simulink model "RunningLEDExample"  (R2015a)
settings: Solver=ode3  SolverMode=SingleTasking  StartTime=0.0  StopTime=inf  FixedStep=Ts  RelTol=1e-3
undefined symbols (not defined in the file): Ts
libraries: simulink x1
(part 1 of 2)
settings Model: ExtModeTrigDuration=2  Creator=kkhoo  LastModifiedBy=kkhoo
settings OptimizationCC: OptimizeModelRefInitCode=on  LifeSpan=1
settings DebuggingCC: UnderspecifiedInitializationDetection=Classic  MergeDetectMultiDrivingBlocksExec=none
settings HardwareCC: ProdBitPerInt=16  ProdBitPerPointer=8  ProdIntDivRoundTo=Zero  ProdEndianess=LittleEndian  ProdWordSize=8  ProdHWDeviceType=Atmel->AVR
settings RTWCC: SystemTargetFile=realtime.tlc  GenerateMakefile=off  TemplateMakefile=realtime.tmf  Description=Run on Target Hardware  RTWVerbose=off  CustomSource=src/Engduino.h src/engduino_wrappers.cpp
settings ERTTargetCC: CombineOutputUpdateFcns=off  ExtModeTransport=3  ExtModeMexFile=ext_serial_win32_comm_rtt  ExtModeMexArgs=0 1 9600  ERTSrcFileBannerTemplate=realtime_code_template.cgt  ERTHdrFileBannerTemplate=realtime_code_template.cgt  ERTDataSrcFileTemplate=realtime_code_template.cgt  ERTDataHdrFileTemplate=realtime_code_template.cgt  ERTCustomFileTemplate=realtime_file_process.tlc

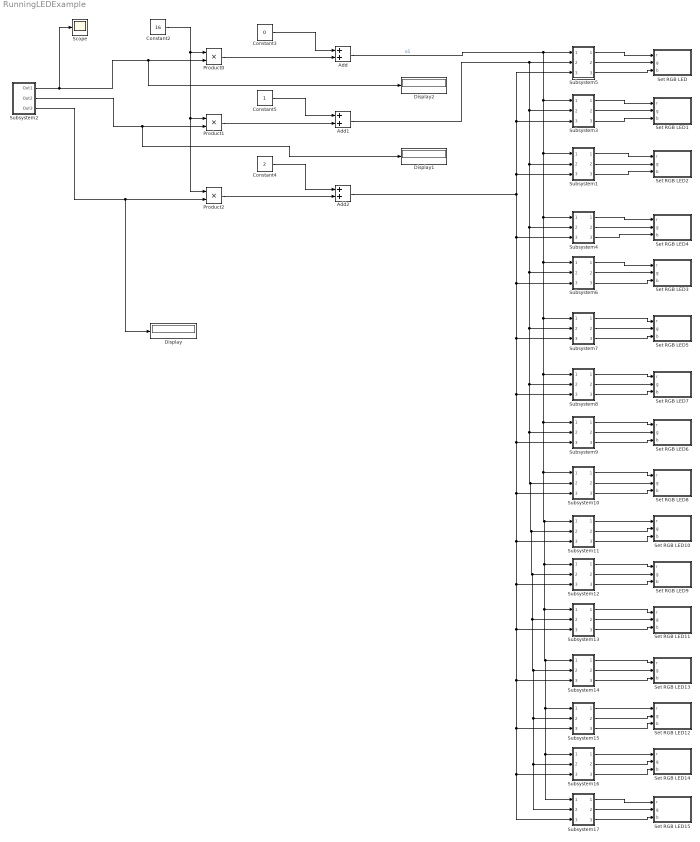
== system RunningLEDExample ==
  Add : Sum  AccumDataTypeStr=single
  Add1 : Sum  AccumDataTypeStr=single
  Add2 : Sum  AccumDataTypeStr=single
  Constant2 : Constant  Value=16  OutDataTypeStr=double
  Constant3 : Constant  Value=0  OutDataTypeStr=single
  Constant4 : Constant  Value=2  OutDataTypeStr=double
  Constant5 : Constant  OutDataTypeStr=double
  Display : Display
  Display1 : Display
  Display2 : Display
  "Product0 " : Product  OutDataTypeStr=double
  Product1 : Product  OutDataTypeStr=double
  Product2 : Product  OutDataTypeStr=double  InputSameDT=on
  Scope : Scope
      settings: YMin=0  YMax=15
  Set RGB LED : MATLAB Function  LoadFcn=|  TreatAsAtomicUnit=on  mask(RGB LED){led_index=0}
      | set_param(gcs, 'CustomSource', strjoin(unique([strsplit(get_param(gcs, 'CustomSource')) ...
      |  'src/engduino_wrappers.cpp' 'src/Engduino.h'])));
      mask prompts: led_index "LED index"
      mask help:
      | Control the Red, Green and Blue color values of the LED specified by the LED index parameter.
      | Both the LED index and the three color values are of type uint8 and must be in the range 0-15.
      settings: AttributesFormatString=LED %<led_index>
  Set RGB LED1 : MATLAB Function  LoadFcn=|  TreatAsAtomicUnit=on  mask(RGB LED){led_index=1}
      | set_param(gcs, 'CustomSource', strjoin(unique([strsplit(get_param(gcs, 'CustomSource')) ...
      |  'src/engduino_wrappers.cpp' 'src/Engduino.h'])));
      mask prompts: led_index "LED index"
      mask help:
      | Control the Red, Green and Blue color values of the LED specified by the LED index parameter.
      | Both the LED index and the three color values are of type uint8 and must be in the range 0-15.
      settings: AttributesFormatString=LED %<led_index>
  Set RGB LED10 : MATLAB Function  LoadFcn=|  TreatAsAtomicUnit=on  mask(RGB LED){led_index=9}
      | set_param(gcs, 'CustomSource', strjoin(unique([strsplit(get_param(gcs, 'CustomSource')) ...
      |  'src/engduino_wrappers.cpp' 'src/Engduino.h'])));
      mask prompts: led_index "LED index"
      mask help:
      | Control the Red, Green and Blue color values of the LED specified by the LED index parameter.
      | Both the LED index and the three color values are of type uint8 and must be in the range 0-15.
      settings: AttributesFormatString=LED %<led_index>
  Set RGB LED11 : MATLAB Function  LoadFcn=|  TreatAsAtomicUnit=on  mask(RGB LED){led_index=11}
      | set_param(gcs, 'CustomSource', strjoin(unique([strsplit(get_param(gcs, 'CustomSource')) ...
      |  'src/engduino_wrappers.cpp' 'src/Engduino.h'])));
      mask prompts: led_index "LED index"
      mask help:
      | Control the Red, Green and Blue color values of the LED specified by the LED index parameter.
      | Both the LED index and the three color values are of type uint8 and must be in the range 0-15.
      settings: AttributesFormatString=LED %<led_index>
  Set RGB LED12 : MATLAB Function  LoadFcn=|  TreatAsAtomicUnit=on  mask(RGB LED){led_index=13}
      | set_param(gcs, 'CustomSource', strjoin(unique([strsplit(get_param(gcs, 'CustomSource')) ...
      |  'src/engduino_wrappers.cpp' 'src/Engduino.h'])));
      mask prompts: led_index "LED index"
      mask help:
      | Control the Red, Green and Blue color values of the LED specified by the LED index parameter.
      | Both the LED index and the three color values are of type uint8 and must be in the range 0-15.
      settings: AttributesFormatString=LED %<led_index>
  Set RGB LED13 : MATLAB Function  LoadFcn=|  TreatAsAtomicUnit=on  mask(RGB LED){led_index=12}
      | set_param(gcs, 'CustomSource', strjoin(unique([strsplit(get_param(gcs, 'CustomSource')) ...
      |  'src/engduino_wrappers.cpp' 'src/Engduino.h'])));
      mask prompts: led_index "LED index"
      mask help:
      | Control the Red, Green and Blue color values of the LED specified by the LED index parameter.
      | Both the LED index and the three color values are of type uint8 and must be in the range 0-15.
      settings: AttributesFormatString=LED %<led_index>
  Set RGB LED14 : MATLAB Function  LoadFcn=|  TreatAsAtomicUnit=on  mask(RGB LED){led_index=14}
      | set_param(gcs, 'CustomSource', strjoin(unique([strsplit(get_param(gcs, 'CustomSource')) ...
      |  'src/engduino_wrappers.cpp' 'src/Engduino.h'])));
      mask prompts: led_index "LED index"
      mask help:
      | Control the Red, Green and Blue color values of the LED specified by the LED index parameter.
      | Both the LED index and the three color values are of type uint8 and must be in the range 0-15.
      settings: AttributesFormatString=LED %<led_index>
  Set RGB LED15 : MATLAB Function  LoadFcn=|  TreatAsAtomicUnit=on  mask(RGB LED){led_index=15}
      | set_param(gcs, 'CustomSource', strjoin(unique([strsplit(get_param(gcs, 'CustomSource')) ...
      |  'src/engduino_wrappers.cpp' 'src/Engduino.h'])));
      mask prompts: led_index "LED index"
      mask help:
      | Control the Red, Green and Blue color values of the LED specified by the LED index parameter.
      | Both the LED index and the three color values are of type uint8 and must be in the range 0-15.
      settings: AttributesFormatString=LED %<led_index>
  Set RGB LED2 : MATLAB Function  LoadFcn=|  TreatAsAtomicUnit=on  mask(RGB LED){led_index=2}
      | set_param(gcs, 'CustomSource', strjoin(unique([strsplit(get_param(gcs, 'CustomSource')) ...
      |  'src/engduino_wrappers.cpp' 'src/Engduino.h'])));
      mask prompts: led_index "LED index"
      mask help:
      | Control the Red, Green and Blue color values of the LED specified by the LED index parameter.
      | Both the LED index and the three color values are of type uint8 and must be in the range 0-15.
      settings: AttributesFormatString=LED %<led_index>
  Set RGB LED3 : MATLAB Function  LoadFcn=|  TreatAsAtomicUnit=on  mask(RGB LED){led_index=4}
      | set_param(gcs, 'CustomSource', strjoin(unique([strsplit(get_param(gcs, 'CustomSource')) ...
      |  'src/engduino_wrappers.cpp' 'src/Engduino.h'])));
      mask prompts: led_index "LED index"
      mask help:
      | Control the Red, Green and Blue color values of the LED specified by the LED index parameter.
      | Both the LED index and the three color values are of type uint8 and must be in the range 0-15.
      settings: AttributesFormatString=LED %<led_index>
  Set RGB LED4 : MATLAB Function  LoadFcn=|  TreatAsAtomicUnit=on  mask(RGB LED){led_index=3}
      | set_param(gcs, 'CustomSource', strjoin(unique([strsplit(get_param(gcs, 'CustomSource')) ...
      |  'src/engduino_wrappers.cpp' 'src/Engduino.h'])));
      mask prompts: led_index "LED index"
      mask help:
      | Control the Red, Green and Blue color values of the LED specified by the LED index parameter.
      | Both the LED index and the three color values are of type uint8 and must be in the range 0-15.
      settings: AttributesFormatString=LED %<led_index>
  Set RGB LED5 : MATLAB Function  LoadFcn=|  TreatAsAtomicUnit=on  mask(RGB LED){led_index=5}
      | set_param(gcs, 'CustomSource', strjoin(unique([strsplit(get_param(gcs, 'CustomSource')) ...
      |  'src/engduino_wrappers.cpp' 'src/Engduino.h'])));
      mask prompts: led_index "LED index"
      mask help:
      | Control the Red, Green and Blue color values of the LED specified by the LED index parameter.
      | Both the LED index and the three color values are of type uint8 and must be in the range 0-15.
      settings: AttributesFormatString=LED %<led_index>
  Set RGB LED6 : MATLAB Function  LoadFcn=|  TreatAsAtomicUnit=on  mask(RGB LED){led_index=7}
      | set_param(gcs, 'CustomSource', strjoin(unique([strsplit(get_param(gcs, 'CustomSource')) ...
      |  'src/engduino_wrappers.cpp' 'src/Engduino.h'])));
      mask prompts: led_index "LED index"
      mask help:
      | Control the Red, Green and Blue color values of the LED specified by the LED index parameter.
      | Both the LED index and the three color values are of type uint8 and must be in the range 0-15.
      settings: AttributesFormatString=LED %<led_index>
  Set RGB LED7 : MATLAB Function  LoadFcn=|  TreatAsAtomicUnit=on  mask(RGB LED){led_index=6}
      | set_param(gcs, 'CustomSource', strjoin(unique([strsplit(get_param(gcs, 'CustomSource')) ...
      |  'src/engduino_wrappers.cpp' 'src/Engduino.h'])));
      mask prompts: led_index "LED index"
      mask help:
      | Control the Red, Green and Blue color values of the LED specified by the LED index parameter.
      | Both the LED index and the three color values are of type uint8 and must be in the range 0-15.
      settings: AttributesFormatString=LED %<led_index>
  Set RGB LED8 : MATLAB Function  LoadFcn=|  TreatAsAtomicUnit=on  mask(RGB LED){led_index=8}
      | set_param(gcs, 'CustomSource', strjoin(unique([strsplit(get_param(gcs, 'CustomSource')) ...
      |  'src/engduino_wrappers.cpp' 'src/Engduino.h'])));
      mask prompts: led_index "LED index"
      mask help:
      | Control the Red, Green and Blue color values of the LED specified by the LED index parameter.
      | Both the LED index and the three color values are of type uint8 and must be in the range 0-15.
      settings: AttributesFormatString=LED %<led_index>
  Set RGB LED9 : MATLAB Function  LoadFcn=|  TreatAsAtomicUnit=on  mask(RGB LED){led_index=10}
      | set_param(gcs, 'CustomSource', strjoin(unique([strsplit(get_param(gcs, 'CustomSource')) ...
      |  'src/engduino_wrappers.cpp' 'src/Engduino.h'])));
      mask prompts: led_index "LED index"
      mask help:
      | Control the Red, Green and Blue color values of the LED specified by the LED index parameter.
      | Both the LED index and the three color values are of type uint8 and must be in the range 0-15.
      settings: AttributesFormatString=LED %<led_index>
  Subsystem1 : Subsystem
  Subsystem10 : Subsystem
  Subsystem11 : Subsystem
  Subsystem12 : Subsystem
  Subsystem13 : Subsystem
  Subsystem14 : Subsystem
  Subsystem15 : Subsystem
  Subsystem16 : Subsystem
  Subsystem17 : Subsystem
  Subsystem2 : Subsystem
  Subsystem3 : Subsystem
  Subsystem4 : Subsystem
  Subsystem5 : Subsystem
  Subsystem6 : Subsystem
  Subsystem7 : Subsystem
  Subsystem8 : Subsystem
  Subsystem9 : Subsystem
  wires:
  Constant2/1 -> "Product0 "/1, Product2/1, Product1/1
  Constant3/1 -> Add/1
  "Product0 "/1 -> Add/2
  Constant5/1 -> Add1/1
  Product1/1 -> Add1/2
  Constant4/1 -> Add2/1
  Product2/1 -> Add2/2
  Subsystem3/1(Out1) -> Set RGB LED1/1(r)
  Subsystem2/1(Out1) -> Scope/1, Display2/1, "Product0 "/2
  Subsystem2/2(Out2) -> Display1/1, Product1/2
  Subsystem2/3(Out3) -> Display/1, Product2/2
  Subsystem5/1(Out1) -> Set RGB LED/1(r)
  Subsystem5/2(Out2) -> Set RGB LED/2(g)
  Subsystem5/3(Out3) -> Set RGB LED/3(b)
  Add/1 -> Subsystem4/1(In1), Subsystem17/1(In1), Subsystem16/1(In1), Subsystem15/1(In1), Subsystem14/1(In1), Subsystem13/1(In1), Subsystem12/1(In1), Subsystem11/1(In1), Subsystem10/1(In1), Subsystem9/1(In1), Subsystem8/1(In1), Subsystem7/1(In1), Subsystem6/1(In1), Subsystem1/1(In1), Subsystem3/1(In1), Subsystem5/1(In1)  "u1"
  Add1/1 -> Subsystem4/2(In2), Subsystem6/2(In2), Subsystem8/2(In2), Subsystem9/2(In2), Subsystem17/2(In2), Subsystem16/2(In2), Subsystem15/2(In2), Subsystem14/2(In2), Subsystem13/2(In2), Subsystem12/2(In2), Subsystem11/2(In2), Subsystem10/2(In2), Subsystem7/2(In2), Subsystem1/2(In2), Subsystem3/2(In2), Subsystem5/2(In2)
  Add2/1 -> Subsystem5/3(In3), Subsystem3/3(In3), Subsystem1/3(In3), Subsystem9/3(In3), Subsystem17/3(In3), Subsystem16/3(In3), Subsystem15/3(In3), Subsystem14/3(In3), Subsystem13/3(In3), Subsystem12/3(In3), Subsystem11/3(In3), Subsystem10/3(In3), Subsystem8/3(In3), Subsystem7/3(In3), Subsystem6/3(In3), Subsystem4/3(In3)
  Subsystem3/2(Out2) -> Set RGB LED1/2(g)
  Subsystem3/3(Out3) -> Set RGB LED1/3(b)
  Subsystem4/1(Out1) -> Set RGB LED4/1(r)
  Subsystem4/2(Out2) -> Set RGB LED4/2(g)
  Subsystem4/3(Out3) -> Set RGB LED4/3(b)
  Subsystem6/1(Out1) -> Set RGB LED3/1(r)
  Subsystem6/2(Out2) -> Set RGB LED3/2(g)
  Subsystem6/3(Out3) -> Set RGB LED3/3(b)
  Subsystem7/1(Out1) -> Set RGB LED5/1(r)
  Subsystem7/2(Out2) -> Set RGB LED5/2(g)
  Subsystem7/3(Out3) -> Set RGB LED5/3(b)
  Subsystem8/1(Out1) -> Set RGB LED7/1(r)
  Subsystem8/2(Out2) -> Set RGB LED7/2(g)
  Subsystem8/3(Out3) -> Set RGB LED7/3(b)
  Subsystem1/1(Out1) -> Set RGB LED2/1(r)
  Subsystem1/2(Out2) -> Set RGB LED2/2(g)
  Subsystem1/3(Out3) -> Set RGB LED2/3(b)
  Subsystem9/1(Out1) -> Set RGB LED6/1(r)
  Subsystem9/2(Out2) -> Set RGB LED6/2(g)
  Subsystem9/3(Out3) -> Set RGB LED6/3(b)
  Subsystem10/1(Out1) -> Set RGB LED8/1(r)
  Subsystem10/2(Out2) -> Set RGB LED8/2(g)
  Subsystem10/3(Out3) -> Set RGB LED8/3(b)
  Subsystem11/1(Out1) -> Set RGB LED10/1(r)
  Subsystem11/2(Out2) -> Set RGB LED10/2(g)
  Subsystem11/3(Out3) -> Set RGB LED10/3(b)
  Subsystem12/1(Out1) -> Set RGB LED9/1(r)
  Subsystem12/2(Out2) -> Set RGB LED9/2(g)
  Subsystem12/3(Out3) -> Set RGB LED9/3(b)
  Subsystem13/1(Out1) -> Set RGB LED11/1(r)
  Subsystem13/2(Out2) -> Set RGB LED11/2(g)
  Subsystem13/3(Out3) -> Set RGB LED11/3(b)
  Subsystem14/2(Out2) -> Set RGB LED13/2(g)
  Subsystem14/1(Out1) -> Set RGB LED13/1(r)
  Subsystem14/3(Out3) -> Set RGB LED13/3(b)
  Subsystem15/1(Out1) -> Set RGB LED12/1(r)
  Subsystem15/2(Out2) -> Set RGB LED12/2(g)
  Subsystem15/3(Out3) -> Set RGB LED12/3(b)
  Subsystem16/1(Out1) -> Set RGB LED14/1(r)
  Subsystem16/2(Out2) -> Set RGB LED14/2(g)
  Subsystem16/3(Out3) -> Set RGB LED14/3(b)
  Subsystem17/1(Out1) -> Set RGB LED15/1(r)
  Subsystem17/2(Out2) -> Set RGB LED15/2(g)
  Subsystem17/3(Out3) -> Set RGB LED15/3(b)

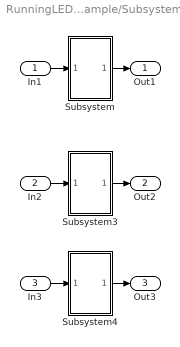
== system RunningLEDExample/Subsystem1 ==
  In1 : Inport
  In2 : Inport  Port=2
  In3 : Inport  Port=3
  Subsystem : Subsystem
  Subsystem3 : Subsystem
  Subsystem4 : Subsystem
  Out1 : Outport
  Out2 : Outport  Port=2
  Out3 : Outport  Port=3
  wires:
  In1/1 -> Subsystem/1(In1)
  Subsystem4/1(Out1) -> Out3/1
  In2/1 -> Subsystem3/1(In1)
  Subsystem/1(Out1) -> Out1/1
  In3/1 -> Subsystem4/1(In1)
  Subsystem3/1(Out1) -> Out2/1

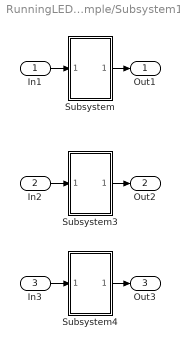
== system RunningLEDExample/Subsystem10 ==
  In1 : Inport
  In2 : Inport  Port=2
  In3 : Inport  Port=3
  Subsystem : Subsystem
  Subsystem3 : Subsystem
  Subsystem4 : Subsystem
  Out1 : Outport
  Out2 : Outport  Port=2
  Out3 : Outport  Port=3
  wires:
  In1/1 -> Subsystem/1(In1)
  Subsystem4/1(Out1) -> Out3/1
  In2/1 -> Subsystem3/1(In1)
  Subsystem/1(Out1) -> Out1/1
  In3/1 -> Subsystem4/1(In1)
  Subsystem3/1(Out1) -> Out2/1

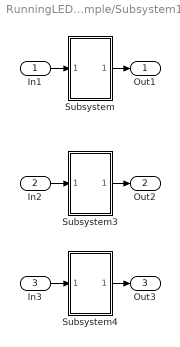
== system RunningLEDExample/Subsystem11 ==
  In1 : Inport
  In2 : Inport  Port=2
  In3 : Inport  Port=3
  Subsystem : Subsystem
  Subsystem3 : Subsystem
  Subsystem4 : Subsystem
  Out1 : Outport
  Out2 : Outport  Port=2
  Out3 : Outport  Port=3
  wires:
  In1/1 -> Subsystem/1(In1)
  Subsystem4/1(Out1) -> Out3/1
  In2/1 -> Subsystem3/1(In1)
  Subsystem/1(Out1) -> Out1/1
  In3/1 -> Subsystem4/1(In1)
  Subsystem3/1(Out1) -> Out2/1

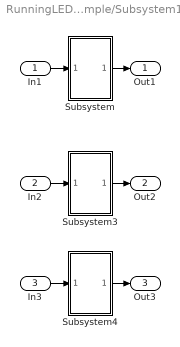
== system RunningLEDExample/Subsystem12 ==
  In1 : Inport
  In2 : Inport  Port=2
  In3 : Inport  Port=3
  Subsystem : Subsystem
  Subsystem3 : Subsystem
  Subsystem4 : Subsystem
  Out1 : Outport
  Out2 : Outport  Port=2
  Out3 : Outport  Port=3
  wires:
  In1/1 -> Subsystem/1(In1)
  Subsystem4/1(Out1) -> Out3/1
  In2/1 -> Subsystem3/1(In1)
  Subsystem/1(Out1) -> Out1/1
  In3/1 -> Subsystem4/1(In1)
  Subsystem3/1(Out1) -> Out2/1

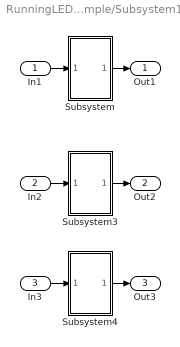
== system RunningLEDExample/Subsystem13 ==
  In1 : Inport
  In2 : Inport  Port=2
  In3 : Inport  Port=3
  Subsystem : Subsystem
  Subsystem3 : Subsystem
  Subsystem4 : Subsystem
  Out1 : Outport
  Out2 : Outport  Port=2
  Out3 : Outport  Port=3
  wires:
  In1/1 -> Subsystem/1(In1)
  Subsystem4/1(Out1) -> Out3/1
  In2/1 -> Subsystem3/1(In1)
  Subsystem/1(Out1) -> Out1/1
  In3/1 -> Subsystem4/1(In1)
  Subsystem3/1(Out1) -> Out2/1

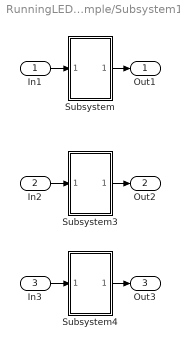
== system RunningLEDExample/Subsystem14 ==
  In1 : Inport
  In2 : Inport  Port=2
  In3 : Inport  Port=3
  Subsystem : Subsystem
  Subsystem3 : Subsystem
  Subsystem4 : Subsystem
  Out1 : Outport
  Out2 : Outport  Port=2
  Out3 : Outport  Port=3
  wires:
  In1/1 -> Subsystem/1(In1)
  Subsystem4/1(Out1) -> Out3/1
  In2/1 -> Subsystem3/1(In1)
  Subsystem/1(Out1) -> Out1/1
  In3/1 -> Subsystem4/1(In1)
  Subsystem3/1(Out1) -> Out2/1

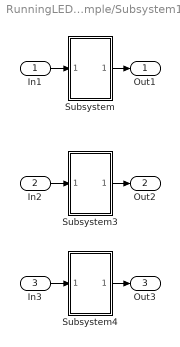
== system RunningLEDExample/Subsystem15 ==
  In1 : Inport
  In2 : Inport  Port=2
  In3 : Inport  Port=3
  Subsystem : Subsystem
  Subsystem3 : Subsystem
  Subsystem4 : Subsystem
  Out1 : Outport
  Out2 : Outport  Port=2
  Out3 : Outport  Port=3
  wires:
  In1/1 -> Subsystem/1(In1)
  Subsystem4/1(Out1) -> Out3/1
  In2/1 -> Subsystem3/1(In1)
  Subsystem/1(Out1) -> Out1/1
  In3/1 -> Subsystem4/1(In1)
  Subsystem3/1(Out1) -> Out2/1

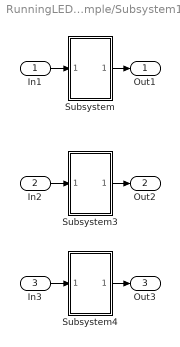
== system RunningLEDExample/Subsystem16 ==
  In1 : Inport
  In2 : Inport  Port=2
  In3 : Inport  Port=3
  Subsystem : Subsystem
  Subsystem3 : Subsystem
  Subsystem4 : Subsystem
  Out1 : Outport
  Out2 : Outport  Port=2
  Out3 : Outport  Port=3
  wires:
  In1/1 -> Subsystem/1(In1)
  Subsystem4/1(Out1) -> Out3/1
  In2/1 -> Subsystem3/1(In1)
  Subsystem/1(Out1) -> Out1/1
  In3/1 -> Subsystem4/1(In1)
  Subsystem3/1(Out1) -> Out2/1

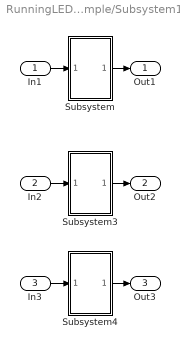
== system RunningLEDExample/Subsystem17 ==
  In1 : Inport
  In2 : Inport  Port=2
  In3 : Inport  Port=3
  Subsystem : Subsystem
  Subsystem3 : Subsystem
  Subsystem4 : Subsystem
  Out1 : Outport
  Out2 : Outport  Port=2
  Out3 : Outport  Port=3
  wires:
  In1/1 -> Subsystem/1(In1)
  Subsystem4/1(Out1) -> Out3/1
  In2/1 -> Subsystem3/1(In1)
  Subsystem/1(Out1) -> Out1/1
  In3/1 -> Subsystem4/1(In1)
  Subsystem3/1(Out1) -> Out2/1

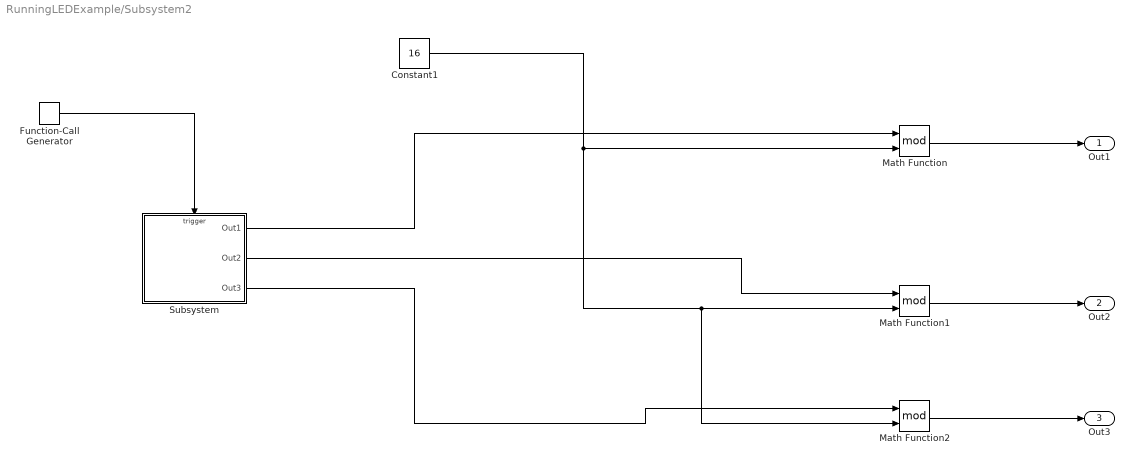
== system RunningLEDExample/Subsystem2 ==
  Constant1 : Constant  Value=16
  Function-Call Generator : simulink/Ports & Subsystems/Function-Call Generator  sample_time=Ts*5  numberOfIterations=1
  Math Function : Math  Operator=mod  SaturateOnIntegerOverflow=on
  Math Function1 : Math  Operator=mod  SaturateOnIntegerOverflow=on
  Math Function2 : Math  Operator=mod  SaturateOnIntegerOverflow=on
  Subsystem : Subsystem
  Out1 : Outport
  Out2 : Outport  Port=2
  Out3 : Outport  Port=3
  wires:
  Math Function/1 -> Out1/1
  Math Function2/1 -> Out3/1
  Math Function1/1 -> Out2/1
  Constant1/1 -> Math Function/2, Math Function2/2, Math Function1/2
  Subsystem/1(Out1) -> Math Function/1
  Subsystem/2(Out2) -> Math Function1/1
  Subsystem/3(Out3) -> Math Function2/1
  Function-Call Generator/1 -> Subsystem/Trigger

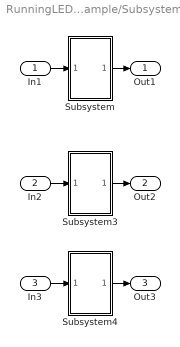
== system RunningLEDExample/Subsystem3 ==
  In1 : Inport
  In2 : Inport  Port=2
  In3 : Inport  Port=3
  Subsystem : Subsystem
  Subsystem3 : Subsystem
  Subsystem4 : Subsystem
  Out1 : Outport
  Out2 : Outport  Port=2
  Out3 : Outport  Port=3
  wires:
  In1/1 -> Subsystem/1(In1)
  Subsystem4/1(Out1) -> Out3/1
  In2/1 -> Subsystem3/1(In1)
  Subsystem/1(Out1) -> Out1/1
  In3/1 -> Subsystem4/1(In1)
  Subsystem3/1(Out1) -> Out2/1

== system RunningLEDExample/Subsystem4 ==
  In1 : Inport
  In2 : Inport  Port=2
  In3 : Inport  Port=3
  Subsystem : Subsystem
  Subsystem3 : Subsystem
  Subsystem4 : Subsystem
  Out1 : Outport
  Out2 : Outport  Port=2
  Out3 : Outport  Port=3
  wires:
  In1/1 -> Subsystem/1(In1)
  Subsystem4/1(Out1) -> Out3/1
  In2/1 -> Subsystem3/1(In1)
  Subsystem/1(Out1) -> Out1/1
  In3/1 -> Subsystem4/1(In1)
  Subsystem3/1(Out1) -> Out2/1

== system RunningLEDExample/Subsystem5 ==
  In1 : Inport
  In2 : Inport  Port=2
  In3 : Inport  Port=3
  Subsystem : Subsystem
  Subsystem3 : Subsystem
  Subsystem4 : Subsystem
  Out1 : Outport
  Out2 : Outport  Port=2
  Out3 : Outport  Port=3
  wires:
  In1/1 -> Subsystem/1(In1)
  Subsystem4/1(Out1) -> Out3/1
  In2/1 -> Subsystem3/1(In1)
  Subsystem/1(Out1) -> Out1/1
  In3/1 -> Subsystem4/1(In1)
  Subsystem3/1(Out1) -> Out2/1

== system RunningLEDExample/Subsystem6 ==
  In1 : Inport
  In2 : Inport  Port=2
  In3 : Inport  Port=3
  Subsystem : Subsystem
  Subsystem3 : Subsystem
  Subsystem4 : Subsystem
  Out1 : Outport
  Out2 : Outport  Port=2
  Out3 : Outport  Port=3
  wires:
  In1/1 -> Subsystem/1(In1)
  Subsystem4/1(Out1) -> Out3/1
  In2/1 -> Subsystem3/1(In1)
  Subsystem/1(Out1) -> Out1/1
  In3/1 -> Subsystem4/1(In1)
  Subsystem3/1(Out1) -> Out2/1

== system RunningLEDExample/Subsystem7 ==
  In1 : Inport
  In2 : Inport  Port=2
  In3 : Inport  Port=3
  Subsystem : Subsystem
  Subsystem3 : Subsystem
  Subsystem4 : Subsystem
  Out1 : Outport
  Out2 : Outport  Port=2
  Out3 : Outport  Port=3
  wires:
  In1/1 -> Subsystem/1(In1)
  Subsystem4/1(Out1) -> Out3/1
  In2/1 -> Subsystem3/1(In1)
  Subsystem/1(Out1) -> Out1/1
  In3/1 -> Subsystem4/1(In1)
  Subsystem3/1(Out1) -> Out2/1

== system RunningLEDExample/Subsystem8 ==
  In1 : Inport
  In2 : Inport  Port=2
  In3 : Inport  Port=3
  Subsystem : Subsystem
  Subsystem3 : Subsystem
  Subsystem4 : Subsystem
  Out1 : Outport
  Out2 : Outport  Port=2
  Out3 : Outport  Port=3
  wires:
  In1/1 -> Subsystem/1(In1)
  Subsystem4/1(Out1) -> Out3/1
  In2/1 -> Subsystem3/1(In1)
  Subsystem/1(Out1) -> Out1/1
  In3/1 -> Subsystem4/1(In1)
  Subsystem3/1(Out1) -> Out2/1

== system RunningLEDExample/Subsystem9 ==
  In1 : Inport
  In2 : Inport  Port=2
  In3 : Inport  Port=3
  Subsystem : Subsystem
  Subsystem3 : Subsystem
  Subsystem4 : Subsystem
  Out1 : Outport
  Out2 : Outport  Port=2
  Out3 : Outport  Port=3
  wires:
  In1/1 -> Subsystem/1(In1)
  Subsystem4/1(Out1) -> Out3/1
  In2/1 -> Subsystem3/1(In1)
  Subsystem/1(Out1) -> Out1/1
  In3/1 -> Subsystem4/1(In1)
  Subsystem3/1(Out1) -> Out2/1

== system RunningLEDExample/Subsystem1/Subsystem ==
  In1 : Inport
  Constant4 : Constant  Value=15  OutDataTypeStr=uint8
  Constant5 : Constant  Value=0  OutDataTypeStr=uint8
  If : If  IfExpression=u1 == 32
  If Action Subsystem : Subsystem  TreatAsAtomicUnit=on
  If Action Subsystem1 : Subsystem  TreatAsAtomicUnit=on
  Merge : Merge
  Out1 : Outport  OutDataTypeStr=uint8
  wires:
  If/1 -> If Action Subsystem/Action
  If/2 -> If Action Subsystem1/Action
  In1/1 -> If/1
  Constant5/1 -> If Action Subsystem1/1(In1)
  Merge/1 -> Out1/1
  Constant4/1 -> If Action Subsystem/1(In1)
  If Action Subsystem/1(Out1) -> Merge/1
  If Action Subsystem1/1(Out1) -> Merge/2

== system RunningLEDExample/Subsystem1/Subsystem3 ==
  In1 : Inport
  Constant4 : Constant  Value=15  OutDataTypeStr=uint8
  Constant5 : Constant  Value=0  OutDataTypeStr=uint8
  If : If  IfExpression=u1 == 33
  If Action Subsystem : Subsystem  TreatAsAtomicUnit=on
  If Action Subsystem1 : Subsystem  TreatAsAtomicUnit=on
  Merge : Merge
  Out1 : Outport  OutDataTypeStr=uint8
  wires:
  If/1 -> If Action Subsystem/Action
  If/2 -> If Action Subsystem1/Action
  In1/1 -> If/1
  Constant5/1 -> If Action Subsystem1/1(In1)
  Merge/1 -> Out1/1
  Constant4/1 -> If Action Subsystem/1(In1)
  If Action Subsystem/1(Out1) -> Merge/1
  If Action Subsystem1/1(Out1) -> Merge/2

== system RunningLEDExample/Subsystem1/Subsystem4 ==
  In1 : Inport
  Constant4 : Constant  Value=15  OutDataTypeStr=uint8
  Constant5 : Constant  Value=0  OutDataTypeStr=uint8
  If : If  IfExpression=u1 == 34
  If Action Subsystem : Subsystem  TreatAsAtomicUnit=on
  If Action Subsystem1 : Subsystem  TreatAsAtomicUnit=on
  Merge : Merge
  Out1 : Outport  OutDataTypeStr=uint8
  wires:
  If/1 -> If Action Subsystem/Action
  If/2 -> If Action Subsystem1/Action
  In1/1 -> If/1
  Constant5/1 -> If Action Subsystem1/1(In1)
  Merge/1 -> Out1/1
  Constant4/1 -> If Action Subsystem/1(In1)
  If Action Subsystem/1(Out1) -> Merge/1
  If Action Subsystem1/1(Out1) -> Merge/2

== system RunningLEDExample/Subsystem10/Subsystem ==
  In1 : Inport
  Constant4 : Constant  Value=15  OutDataTypeStr=uint8
  Constant5 : Constant  Value=0  OutDataTypeStr=uint8
  If : If  IfExpression=u1 == 128
  If Action Subsystem : Subsystem  TreatAsAtomicUnit=on
  If Action Subsystem1 : Subsystem  TreatAsAtomicUnit=on
  Merge : Merge
  Out1 : Outport  OutDataTypeStr=uint8
  wires:
  If/1 -> If Action Subsystem/Action
  If/2 -> If Action Subsystem1/Action
  In1/1 -> If/1
  Constant5/1 -> If Action Subsystem1/1(In1)
  Merge/1 -> Out1/1
  Constant4/1 -> If Action Subsystem/1(In1)
  If Action Subsystem/1(Out1) -> Merge/1
  If Action Subsystem1/1(Out1) -> Merge/2

== system RunningLEDExample/Subsystem10/Subsystem3 ==
  In1 : Inport
  Constant4 : Constant  Value=15  OutDataTypeStr=uint8
  Constant5 : Constant  Value=0  OutDataTypeStr=uint8
  If : If  IfExpression=u1 == 129
  If Action Subsystem : Subsystem  TreatAsAtomicUnit=on
  If Action Subsystem1 : Subsystem  TreatAsAtomicUnit=on
  Merge : Merge
  Out1 : Outport  OutDataTypeStr=uint8
  wires:
  If/1 -> If Action Subsystem/Action
  If/2 -> If Action Subsystem1/Action
  In1/1 -> If/1
  Constant5/1 -> If Action Subsystem1/1(In1)
  Merge/1 -> Out1/1
  Constant4/1 -> If Action Subsystem/1(In1)
  If Action Subsystem/1(Out1) -> Merge/1
  If Action Subsystem1/1(Out1) -> Merge/2

== system RunningLEDExample/Subsystem10/Subsystem4 ==
  In1 : Inport
  Constant4 : Constant  Value=15  OutDataTypeStr=uint8
  Constant5 : Constant  Value=0  OutDataTypeStr=uint8
  If : If  IfExpression=u1 == 130
  If Action Subsystem : Subsystem  TreatAsAtomicUnit=on
  If Action Subsystem1 : Subsystem  TreatAsAtomicUnit=on
  Merge : Merge
  Out1 : Outport  OutDataTypeStr=uint8
  wires:
  If/1 -> If Action Subsystem/Action
  If/2 -> If Action Subsystem1/Action
  In1/1 -> If/1
  Constant5/1 -> If Action Subsystem1/1(In1)
  Merge/1 -> Out1/1
  Constant4/1 -> If Action Subsystem/1(In1)
  If Action Subsystem/1(Out1) -> Merge/1
  If Action Subsystem1/1(Out1) -> Merge/2

== system RunningLEDExample/Subsystem11/Subsystem ==
  In1 : Inport
  Constant4 : Constant  Value=15  OutDataTypeStr=uint8
  Constant5 : Constant  Value=0  OutDataTypeStr=uint8
  If : If  IfExpression=u1 == 144
  If Action Subsystem : Subsystem  TreatAsAtomicUnit=on
  If Action Subsystem1 : Subsystem  TreatAsAtomicUnit=on
  Merge : Merge
  Out1 : Outport  OutDataTypeStr=uint8
  wires:
  If/1 -> If Action Subsystem/Action
  If/2 -> If Action Subsystem1/Action
  In1/1 -> If/1
  Constant5/1 -> If Action Subsystem1/1(In1)
  Merge/1 -> Out1/1
  Constant4/1 -> If Action Subsystem/1(In1)
  If Action Subsystem/1(Out1) -> Merge/1
  If Action Subsystem1/1(Out1) -> Merge/2

== system RunningLEDExample/Subsystem11/Subsystem3 ==
  In1 : Inport
  Constant4 : Constant  Value=15  OutDataTypeStr=uint8
  Constant5 : Constant  Value=0  OutDataTypeStr=uint8
  If : If  IfExpression=u1 == 145
  If Action Subsystem : Subsystem  TreatAsAtomicUnit=on
  If Action Subsystem1 : Subsystem  TreatAsAtomicUnit=on
  Merge : Merge
  Out1 : Outport  OutDataTypeStr=uint8
  wires:
  If/1 -> If Action Subsystem/Action
  If/2 -> If Action Subsystem1/Action
  In1/1 -> If/1
  Constant5/1 -> If Action Subsystem1/1(In1)
  Merge/1 -> Out1/1
  Constant4/1 -> If Action Subsystem/1(In1)
  If Action Subsystem/1(Out1) -> Merge/1
  If Action Subsystem1/1(Out1) -> Merge/2

== system RunningLEDExample/Subsystem11/Subsystem4 ==
  In1 : Inport
  Constant4 : Constant  Value=15  OutDataTypeStr=uint8
  Constant5 : Constant  Value=0  OutDataTypeStr=uint8
  If : If  IfExpression=u1 == 146
  If Action Subsystem : Subsystem  TreatAsAtomicUnit=on
  If Action Subsystem1 : Subsystem  TreatAsAtomicUnit=on
  Merge : Merge
  Out1 : Outport  OutDataTypeStr=uint8
  wires:
  If/1 -> If Action Subsystem/Action
  If/2 -> If Action Subsystem1/Action
  In1/1 -> If/1
  Constant5/1 -> If Action Subsystem1/1(In1)
  Merge/1 -> Out1/1
  Constant4/1 -> If Action Subsystem/1(In1)
  If Action Subsystem/1(Out1) -> Merge/1
  If Action Subsystem1/1(Out1) -> Merge/2

== system RunningLEDExample/Subsystem12/Subsystem ==
  In1 : Inport
  Constant4 : Constant  Value=15  OutDataTypeStr=uint8
  Constant5 : Constant  Value=0  OutDataTypeStr=uint8
  If : If  IfExpression=u1 == 160
  If Action Subsystem : Subsystem  TreatAsAtomicUnit=on
  If Action Subsystem1 : Subsystem  TreatAsAtomicUnit=on
  Merge : Merge
  Out1 : Outport  OutDataTypeStr=uint8
  wires:
  If/1 -> If Action Subsystem/Action
  If/2 -> If Action Subsystem1/Action
  In1/1 -> If/1
  Constant5/1 -> If Action Subsystem1/1(In1)
  Merge/1 -> Out1/1
  Constant4/1 -> If Action Subsystem/1(In1)
  If Action Subsystem/1(Out1) -> Merge/1
  If Action Subsystem1/1(Out1) -> Merge/2

== system RunningLEDExample/Subsystem12/Subsystem3 ==
  In1 : Inport
  Constant4 : Constant  Value=15  OutDataTypeStr=uint8
  Constant5 : Constant  Value=0  OutDataTypeStr=uint8
  If : If  IfExpression=u1 == 161
  If Action Subsystem : Subsystem  TreatAsAtomicUnit=on
  If Action Subsystem1 : Subsystem  TreatAsAtomicUnit=on
  Merge : Merge
  Out1 : Outport  OutDataTypeStr=uint8
  wires:
  If/1 -> If Action Subsystem/Action
  If/2 -> If Action Subsystem1/Action
  In1/1 -> If/1
  Constant5/1 -> If Action Subsystem1/1(In1)
  Merge/1 -> Out1/1
  Constant4/1 -> If Action Subsystem/1(In1)
  If Action Subsystem/1(Out1) -> Merge/1
  If Action Subsystem1/1(Out1) -> Merge/2

== system RunningLEDExample/Subsystem12/Subsystem4 ==
  In1 : Inport
  Constant4 : Constant  Value=15  OutDataTypeStr=uint8
  Constant5 : Constant  Value=0  OutDataTypeStr=uint8
  If : If  IfExpression=u1 == 162
  If Action Subsystem : Subsystem  TreatAsAtomicUnit=on
  If Action Subsystem1 : Subsystem  TreatAsAtomicUnit=on
  Merge : Merge
  Out1 : Outport  OutDataTypeStr=uint8
  wires:
  If/1 -> If Action Subsystem/Action
  If/2 -> If Action Subsystem1/Action
  In1/1 -> If/1
  Constant5/1 -> If Action Subsystem1/1(In1)
  Merge/1 -> Out1/1
  Constant4/1 -> If Action Subsystem/1(In1)
  If Action Subsystem/1(Out1) -> Merge/1
  If Action Subsystem1/1(Out1) -> Merge/2

== system RunningLEDExample/Subsystem13/Subsystem ==
  In1 : Inport
  Constant4 : Constant  Value=15  OutDataTypeStr=uint8
  Constant5 : Constant  Value=0  OutDataTypeStr=uint8
  If : If  IfExpression=u1 == 176
  If Action Subsystem : Subsystem  TreatAsAtomicUnit=on
  If Action Subsystem1 : Subsystem  TreatAsAtomicUnit=on
  Merge : Merge
  Out1 : Outport  OutDataTypeStr=uint8
  wires:
  If/1 -> If Action Subsystem/Action
  If/2 -> If Action Subsystem1/Action
  In1/1 -> If/1
  Constant5/1 -> If Action Subsystem1/1(In1)
  Merge/1 -> Out1/1
  Constant4/1 -> If Action Subsystem/1(In1)
  If Action Subsystem/1(Out1) -> Merge/1
  If Action Subsystem1/1(Out1) -> Merge/2

== system RunningLEDExample/Subsystem13/Subsystem3 ==
  In1 : Inport
  Constant4 : Constant  Value=15  OutDataTypeStr=uint8
  Constant5 : Constant  Value=0  OutDataTypeStr=uint8
  If : If  IfExpression=u1 == 177
  If Action Subsystem : Subsystem  TreatAsAtomicUnit=on
  If Action Subsystem1 : Subsystem  TreatAsAtomicUnit=on
  Merge : Merge
  Out1 : Outport  OutDataTypeStr=uint8
  wires:
  If/1 -> If Action Subsystem/Action
  If/2 -> If Action Subsystem1/Action
  In1/1 -> If/1
  Constant5/1 -> If Action Subsystem1/1(In1)
  Merge/1 -> Out1/1
  Constant4/1 -> If Action Subsystem/1(In1)
  If Action Subsystem/1(Out1) -> Merge/1
  If Action Subsystem1/1(Out1) -> Merge/2

== system RunningLEDExample/Subsystem13/Subsystem4 ==
  In1 : Inport
  Constant4 : Constant  Value=15  OutDataTypeStr=uint8
  Constant5 : Constant  Value=0  OutDataTypeStr=uint8
  If : If  IfExpression=u1 == 178
  If Action Subsystem : Subsystem  TreatAsAtomicUnit=on
  If Action Subsystem1 : Subsystem  TreatAsAtomicUnit=on
  Merge : Merge
  Out1 : Outport  OutDataTypeStr=uint8
  wires:
  If/1 -> If Action Subsystem/Action
  If/2 -> If Action Subsystem1/Action
  In1/1 -> If/1
  Constant5/1 -> If Action Subsystem1/1(In1)
  Merge/1 -> Out1/1
  Constant4/1 -> If Action Subsystem/1(In1)
  If Action Subsystem/1(Out1) -> Merge/1
  If Action Subsystem1/1(Out1) -> Merge/2

== system RunningLEDExample/Subsystem14/Subsystem ==
  In1 : Inport
  Constant4 : Constant  Value=15  OutDataTypeStr=uint8
  Constant5 : Constant  Value=0  OutDataTypeStr=uint8
  If : If  IfExpression=u1 == 192
  If Action Subsystem : Subsystem  TreatAsAtomicUnit=on
  If Action Subsystem1 : Subsystem  TreatAsAtomicUnit=on
  Merge : Merge
  Out1 : Outport  OutDataTypeStr=uint8
  wires:
  If/1 -> If Action Subsystem/Action
  If/2 -> If Action Subsystem1/Action
  In1/1 -> If/1
  Constant5/1 -> If Action Subsystem1/1(In1)
  Merge/1 -> Out1/1
  Constant4/1 -> If Action Subsystem/1(In1)
  If Action Subsystem/1(Out1) -> Merge/1
  If Action Subsystem1/1(Out1) -> Merge/2

== system RunningLEDExample/Subsystem14/Subsystem3 ==
  In1 : Inport
  Constant4 : Constant  Value=15  OutDataTypeStr=uint8
  Constant5 : Constant  Value=0  OutDataTypeStr=uint8
  If : If  IfExpression=u1 == 193
  If Action Subsystem : Subsystem  TreatAsAtomicUnit=on
  If Action Subsystem1 : Subsystem  TreatAsAtomicUnit=on
  Merge : Merge
  Out1 : Outport  OutDataTypeStr=uint8
  wires:
  If/1 -> If Action Subsystem/Action
  If/2 -> If Action Subsystem1/Action
  In1/1 -> If/1
  Constant5/1 -> If Action Subsystem1/1(In1)
  Merge/1 -> Out1/1
  Constant4/1 -> If Action Subsystem/1(In1)
  If Action Subsystem/1(Out1) -> Merge/1
  If Action Subsystem1/1(Out1) -> Merge/2

== system RunningLEDExample/Subsystem14/Subsystem4 ==
  In1 : Inport
  Constant4 : Constant  Value=15  OutDataTypeStr=uint8
  Constant5 : Constant  Value=0  OutDataTypeStr=uint8
  If : If  IfExpression=u1 == 194
  If Action Subsystem : Subsystem  TreatAsAtomicUnit=on
  If Action Subsystem1 : Subsystem  TreatAsAtomicUnit=on
  Merge : Merge
  Out1 : Outport  OutDataTypeStr=uint8
  wires:
  If/1 -> If Action Subsystem/Action
  If/2 -> If Action Subsystem1/Action
  In1/1 -> If/1
  Constant5/1 -> If Action Subsystem1/1(In1)
  Merge/1 -> Out1/1
  Constant4/1 -> If Action Subsystem/1(In1)
  If Action Subsystem/1(Out1) -> Merge/1
  If Action Subsystem1/1(Out1) -> Merge/2

== system RunningLEDExample/Subsystem15/Subsystem ==
  In1 : Inport
  Constant4 : Constant  Value=15  OutDataTypeStr=uint8
  Constant5 : Constant  Value=0  OutDataTypeStr=uint8
  If : If  IfExpression=u1 == 208
  If Action Subsystem : Subsystem  TreatAsAtomicUnit=on
  If Action Subsystem1 : Subsystem  TreatAsAtomicUnit=on
  Merge : Merge
  Out1 : Outport  OutDataTypeStr=uint8
  wires:
  If/1 -> If Action Subsystem/Action
  If/2 -> If Action Subsystem1/Action
  In1/1 -> If/1
  Constant5/1 -> If Action Subsystem1/1(In1)
  Merge/1 -> Out1/1
  Constant4/1 -> If Action Subsystem/1(In1)
  If Action Subsystem/1(Out1) -> Merge/1
  If Action Subsystem1/1(Out1) -> Merge/2

== system RunningLEDExample/Subsystem15/Subsystem3 ==
  In1 : Inport
  Constant4 : Constant  Value=15  OutDataTypeStr=uint8
  Constant5 : Constant  Value=0  OutDataTypeStr=uint8
  If : If  IfExpression=u1 == 209
  If Action Subsystem : Subsystem  TreatAsAtomicUnit=on
  If Action Subsystem1 : Subsystem  TreatAsAtomicUnit=on
  Merge : Merge
  Out1 : Outport  OutDataTypeStr=uint8
  wires:
  If/1 -> If Action Subsystem/Action
  If/2 -> If Action Subsystem1/Action
  In1/1 -> If/1
  Constant5/1 -> If Action Subsystem1/1(In1)
  Merge/1 -> Out1/1
  Constant4/1 -> If Action Subsystem/1(In1)
  If Action Subsystem/1(Out1) -> Merge/1
  If Action Subsystem1/1(Out1) -> Merge/2

== system RunningLEDExample/Subsystem15/Subsystem4 ==
  In1 : Inport
  Constant4 : Constant  Value=15  OutDataTypeStr=uint8
  Constant5 : Constant  Value=0  OutDataTypeStr=uint8
  If : If  IfExpression=u1 == 210
  If Action Subsystem : Subsystem  TreatAsAtomicUnit=on
  If Action Subsystem1 : Subsystem  TreatAsAtomicUnit=on
  Merge : Merge
  Out1 : Outport  OutDataTypeStr=uint8
  wires:
  If/1 -> If Action Subsystem/Action
  If/2 -> If Action Subsystem1/Action
  In1/1 -> If/1
  Constant5/1 -> If Action Subsystem1/1(In1)
  Merge/1 -> Out1/1
  Constant4/1 -> If Action Subsystem/1(In1)
  If Action Subsystem/1(Out1) -> Merge/1
  If Action Subsystem1/1(Out1) -> Merge/2

== system RunningLEDExample/Subsystem16/Subsystem ==
  In1 : Inport
  Constant4 : Constant  Value=15  OutDataTypeStr=uint8
  Constant5 : Constant  Value=0  OutDataTypeStr=uint8
  If : If  IfExpression=u1 == 224
  If Action Subsystem : Subsystem  TreatAsAtomicUnit=on
  If Action Subsystem1 : Subsystem  TreatAsAtomicUnit=on
  Merge : Merge
  Out1 : Outport  OutDataTypeStr=uint8
  wires:
  If/1 -> If Action Subsystem/Action
  If/2 -> If Action Subsystem1/Action
  In1/1 -> If/1
  Constant5/1 -> If Action Subsystem1/1(In1)
  Merge/1 -> Out1/1
  Constant4/1 -> If Action Subsystem/1(In1)
  If Action Subsystem/1(Out1) -> Merge/1
  If Action Subsystem1/1(Out1) -> Merge/2

== system RunningLEDExample/Subsystem16/Subsystem3 ==
  In1 : Inport
  Constant4 : Constant  Value=15  OutDataTypeStr=uint8
  Constant5 : Constant  Value=0  OutDataTypeStr=uint8
  If : If  IfExpression=u1 == 225
  If Action Subsystem : Subsystem  TreatAsAtomicUnit=on
  If Action Subsystem1 : Subsystem  TreatAsAtomicUnit=on
  Merge : Merge
  Out1 : Outport  OutDataTypeStr=uint8
  wires:
  If/1 -> If Action Subsystem/Action
  If/2 -> If Action Subsystem1/Action
  In1/1 -> If/1
  Constant5/1 -> If Action Subsystem1/1(In1)
  Merge/1 -> Out1/1
  Constant4/1 -> If Action Subsystem/1(In1)
  If Action Subsystem/1(Out1) -> Merge/1
  If Action Subsystem1/1(Out1) -> Merge/2

== system RunningLEDExample/Subsystem16/Subsystem4 ==
  In1 : Inport
  Constant4 : Constant  Value=15  OutDataTypeStr=uint8
  Constant5 : Constant  Value=0  OutDataTypeStr=uint8
  If : If  IfExpression=u1 == 226
  If Action Subsystem : Subsystem  TreatAsAtomicUnit=on
  If Action Subsystem1 : Subsystem  TreatAsAtomicUnit=on
  Merge : Merge
  Out1 : Outport  OutDataTypeStr=uint8
  wires:
  If/1 -> If Action Subsystem/Action
  If/2 -> If Action Subsystem1/Action
  In1/1 -> If/1
  Constant5/1 -> If Action Subsystem1/1(In1)
  Merge/1 -> Out1/1
  Constant4/1 -> If Action Subsystem/1(In1)
  If Action Subsystem/1(Out1) -> Merge/1
  If Action Subsystem1/1(Out1) -> Merge/2

== system RunningLEDExample/Subsystem17/Subsystem ==
  In1 : Inport
  Constant4 : Constant  Value=15  OutDataTypeStr=uint8
  Constant5 : Constant  Value=0  OutDataTypeStr=uint8
  If : If  IfExpression=u1 == 240
  If Action Subsystem : Subsystem  TreatAsAtomicUnit=on
  If Action Subsystem1 : Subsystem  TreatAsAtomicUnit=on
  Merge : Merge
  Out1 : Outport  OutDataTypeStr=uint8
  wires:
  If/1 -> If Action Subsystem/Action
  If/2 -> If Action Subsystem1/Action
  In1/1 -> If/1
  Constant5/1 -> If Action Subsystem1/1(In1)
  Merge/1 -> Out1/1
  Constant4/1 -> If Action Subsystem/1(In1)
  If Action Subsystem/1(Out1) -> Merge/1
  If Action Subsystem1/1(Out1) -> Merge/2

== system RunningLEDExample/Subsystem17/Subsystem3 ==
  In1 : Inport
  Constant4 : Constant  Value=15  OutDataTypeStr=uint8
  Constant5 : Constant  Value=0  OutDataTypeStr=uint8
  If : If  IfExpression=u1 == 241
  If Action Subsystem : Subsystem  TreatAsAtomicUnit=on
  If Action Subsystem1 : Subsystem  TreatAsAtomicUnit=on
  Merge : Merge
  Out1 : Outport  OutDataTypeStr=uint8
  wires:
  If/1 -> If Action Subsystem/Action
  If/2 -> If Action Subsystem1/Action
  In1/1 -> If/1
  Constant5/1 -> If Action Subsystem1/1(In1)
  Merge/1 -> Out1/1
  Constant4/1 -> If Action Subsystem/1(In1)
  If Action Subsystem/1(Out1) -> Merge/1
  If Action Subsystem1/1(Out1) -> Merge/2

== system RunningLEDExample/Subsystem17/Subsystem4 ==
  In1 : Inport
  Constant4 : Constant  Value=15  OutDataTypeStr=uint8
  Constant5 : Constant  Value=0  OutDataTypeStr=uint8
  If : If  IfExpression=u1 == 242
  If Action Subsystem : Subsystem  TreatAsAtomicUnit=on
  If Action Subsystem1 : Subsystem  TreatAsAtomicUnit=on
  Merge : Merge
  Out1 : Outport  OutDataTypeStr=uint8
  wires:
  If/1 -> If Action Subsystem/Action
  If/2 -> If Action Subsystem1/Action
  In1/1 -> If/1
  Constant5/1 -> If Action Subsystem1/1(In1)
  Merge/1 -> Out1/1
  Constant4/1 -> If Action Subsystem/1(In1)
  If Action Subsystem/1(Out1) -> Merge/1
  If Action Subsystem1/1(Out1) -> Merge/2

== system RunningLEDExample/Subsystem2/Subsystem ==
  function : TriggerPort  TriggerType=function-call  SampleTimeType=periodic  SampleTime=Ts*5
  Add : Sum
  Constant : Constant
  Unit Delay : UnitDelay  SampleTime=-1
  Unit Delay1 : UnitDelay  SampleTime=-1
  Out1 : Outport
  Out2 : Outport  Port=2
  Out3 : Outport  Port=3
  wires:
  Unit Delay/1 -> Out2/1, Unit Delay1/1, Add/2
  Constant/1 -> Add/1
  Add/1 -> Out1/1, Unit Delay/1
  Unit Delay1/1 -> Out3/1

== system RunningLEDExample/Subsystem3/Subsystem ==
  In1 : Inport
  Constant4 : Constant  Value=15  OutDataTypeStr=uint8
  Constant5 : Constant  Value=0  OutDataTypeStr=uint8
  If : If  IfExpression=u1 == 16
  If Action Subsystem : Subsystem  TreatAsAtomicUnit=on
  If Action Subsystem1 : Subsystem  TreatAsAtomicUnit=on
  Merge : Merge
  Out1 : Outport  OutDataTypeStr=uint8
  wires:
  If/1 -> If Action Subsystem/Action
  If/2 -> If Action Subsystem1/Action
  In1/1 -> If/1
  Constant5/1 -> If Action Subsystem1/1(In1)
  Merge/1 -> Out1/1
  Constant4/1 -> If Action Subsystem/1(In1)
  If Action Subsystem/1(Out1) -> Merge/1
  If Action Subsystem1/1(Out1) -> Merge/2

== system RunningLEDExample/Subsystem3/Subsystem3 ==
  In1 : Inport
  Constant4 : Constant  Value=15  OutDataTypeStr=uint8
  Constant5 : Constant  Value=0  OutDataTypeStr=uint8
  If : If  IfExpression=u1 == 17
  If Action Subsystem : Subsystem  TreatAsAtomicUnit=on
  If Action Subsystem1 : Subsystem  TreatAsAtomicUnit=on
  Merge : Merge
  Out1 : Outport  OutDataTypeStr=uint8
  wires:
  If/1 -> If Action Subsystem/Action
  If/2 -> If Action Subsystem1/Action
  In1/1 -> If/1
  Constant5/1 -> If Action Subsystem1/1(In1)
  Merge/1 -> Out1/1
  Constant4/1 -> If Action Subsystem/1(In1)
  If Action Subsystem/1(Out1) -> Merge/1
  If Action Subsystem1/1(Out1) -> Merge/2

== system RunningLEDExample/Subsystem3/Subsystem4 ==
  In1 : Inport
  Constant4 : Constant  Value=15  OutDataTypeStr=uint8
  Constant5 : Constant  Value=0  OutDataTypeStr=uint8
  If : If  IfExpression=u1 == 18
  If Action Subsystem : Subsystem  TreatAsAtomicUnit=on
  If Action Subsystem1 : Subsystem  TreatAsAtomicUnit=on
  Merge : Merge
  Out1 : Outport  OutDataTypeStr=uint8
  wires:
  If/1 -> If Action Subsystem/Action
  If/2 -> If Action Subsystem1/Action
  In1/1 -> If/1
  Constant5/1 -> If Action Subsystem1/1(In1)
  Merge/1 -> Out1/1
  Constant4/1 -> If Action Subsystem/1(In1)
  If Action Subsystem/1(Out1) -> Merge/1
  If Action Subsystem1/1(Out1) -> Merge/2

== system RunningLEDExample/Subsystem4/Subsystem ==
  In1 : Inport
  Constant4 : Constant  Value=15  OutDataTypeStr=uint8
  Constant5 : Constant  Value=0  OutDataTypeStr=uint8
  If : If  IfExpression=u1 == 48
  If Action Subsystem : Subsystem  TreatAsAtomicUnit=on
  If Action Subsystem1 : Subsystem  TreatAsAtomicUnit=on
  Merge : Merge
  Out1 : Outport  OutDataTypeStr=uint8
  wires:
  If/1 -> If Action Subsystem/Action
  If/2 -> If Action Subsystem1/Action
  In1/1 -> If/1
  Constant5/1 -> If Action Subsystem1/1(In1)
  Merge/1 -> Out1/1
  Constant4/1 -> If Action Subsystem/1(In1)
  If Action Subsystem/1(Out1) -> Merge/1
  If Action Subsystem1/1(Out1) -> Merge/2

== system RunningLEDExample/Subsystem4/Subsystem3 ==
  In1 : Inport
  Constant4 : Constant  Value=15  OutDataTypeStr=uint8
  Constant5 : Constant  Value=0  OutDataTypeStr=uint8
  If : If  IfExpression=u1 == 49
  If Action Subsystem : Subsystem  TreatAsAtomicUnit=on
  If Action Subsystem1 : Subsystem  TreatAsAtomicUnit=on
  Merge : Merge
  Out1 : Outport  OutDataTypeStr=uint8
  wires:
  If/1 -> If Action Subsystem/Action
  If/2 -> If Action Subsystem1/Action
  In1/1 -> If/1
  Constant5/1 -> If Action Subsystem1/1(In1)
  Merge/1 -> Out1/1
  Constant4/1 -> If Action Subsystem/1(In1)
  If Action Subsystem/1(Out1) -> Merge/1
  If Action Subsystem1/1(Out1) -> Merge/2

== system RunningLEDExample/Subsystem4/Subsystem4 ==
  In1 : Inport
  Constant4 : Constant  Value=15  OutDataTypeStr=uint8
  Constant5 : Constant  Value=0  OutDataTypeStr=uint8
  If : If  IfExpression=u1 == 50
  If Action Subsystem : Subsystem  TreatAsAtomicUnit=on
  If Action Subsystem1 : Subsystem  TreatAsAtomicUnit=on
  Merge : Merge
  Out1 : Outport  OutDataTypeStr=uint8
  wires:
  If/1 -> If Action Subsystem/Action
  If/2 -> If Action Subsystem1/Action
  In1/1 -> If/1
  Constant5/1 -> If Action Subsystem1/1(In1)
  Merge/1 -> Out1/1
  Constant4/1 -> If Action Subsystem/1(In1)
  If Action Subsystem/1(Out1) -> Merge/1
  If Action Subsystem1/1(Out1) -> Merge/2

== system RunningLEDExample/Subsystem5/Subsystem ==
  In1 : Inport
  Constant4 : Constant  Value=15  OutDataTypeStr=uint8
  Constant5 : Constant  Value=0  OutDataTypeStr=uint8
  If : If  IfExpression=u1 == 0
  If Action Subsystem : Subsystem  TreatAsAtomicUnit=on
  If Action Subsystem1 : Subsystem  TreatAsAtomicUnit=on
  Merge : Merge
  Out1 : Outport  OutDataTypeStr=uint8
  wires:
  If/1 -> If Action Subsystem/Action
  If/2 -> If Action Subsystem1/Action
  In1/1 -> If/1
  Constant5/1 -> If Action Subsystem1/1(In1)
  Merge/1 -> Out1/1
  Constant4/1 -> If Action Subsystem/1(In1)
  If Action Subsystem/1(Out1) -> Merge/1
  If Action Subsystem1/1(Out1) -> Merge/2

== system RunningLEDExample/Subsystem5/Subsystem3 ==
  In1 : Inport
  Constant4 : Constant  Value=15  OutDataTypeStr=uint8
  Constant5 : Constant  Value=0  OutDataTypeStr=uint8
  If : If  IfExpression=u1 == 1
  If Action Subsystem : Subsystem  TreatAsAtomicUnit=on
  If Action Subsystem1 : Subsystem  TreatAsAtomicUnit=on
  Merge : Merge
  Out1 : Outport  OutDataTypeStr=uint8
  wires:
  If/1 -> If Action Subsystem/Action
  If/2 -> If Action Subsystem1/Action
  In1/1 -> If/1
  Constant5/1 -> If Action Subsystem1/1(In1)
  Merge/1 -> Out1/1
  Constant4/1 -> If Action Subsystem/1(In1)
  If Action Subsystem/1(Out1) -> Merge/1
  If Action Subsystem1/1(Out1) -> Merge/2

== system RunningLEDExample/Subsystem5/Subsystem4 ==
  In1 : Inport
  Constant4 : Constant  Value=15  OutDataTypeStr=uint8
  Constant5 : Constant  Value=0  OutDataTypeStr=uint8
  If : If  IfExpression=u1 == 2
  If Action Subsystem : Subsystem  TreatAsAtomicUnit=on
  If Action Subsystem1 : Subsystem  TreatAsAtomicUnit=on
  Merge : Merge
  Out1 : Outport  OutDataTypeStr=uint8
  wires:
  If/1 -> If Action Subsystem/Action
  If/2 -> If Action Subsystem1/Action
  In1/1 -> If/1
  Constant5/1 -> If Action Subsystem1/1(In1)
  Merge/1 -> Out1/1
  Constant4/1 -> If Action Subsystem/1(In1)
  If Action Subsystem/1(Out1) -> Merge/1
  If Action Subsystem1/1(Out1) -> Merge/2

== system RunningLEDExample/Subsystem6/Subsystem ==
  In1 : Inport
  Constant4 : Constant  Value=15  OutDataTypeStr=uint8
  Constant5 : Constant  Value=0  OutDataTypeStr=uint8
  If : If  IfExpression=u1 == 64
  If Action Subsystem : Subsystem  TreatAsAtomicUnit=on
  If Action Subsystem1 : Subsystem  TreatAsAtomicUnit=on
  Merge : Merge
  Out1 : Outport  OutDataTypeStr=uint8
  wires:
  If/1 -> If Action Subsystem/Action
  If/2 -> If Action Subsystem1/Action
  In1/1 -> If/1
  Constant5/1 -> If Action Subsystem1/1(In1)
  Merge/1 -> Out1/1
  Constant4/1 -> If Action Subsystem/1(In1)
  If Action Subsystem/1(Out1) -> Merge/1
  If Action Subsystem1/1(Out1) -> Merge/2

== system RunningLEDExample/Subsystem6/Subsystem3 ==
  In1 : Inport
  Constant4 : Constant  Value=15  OutDataTypeStr=uint8
  Constant5 : Constant  Value=0  OutDataTypeStr=uint8
  If : If  IfExpression=u1 == 65
  If Action Subsystem : Subsystem  TreatAsAtomicUnit=on
  If Action Subsystem1 : Subsystem  TreatAsAtomicUnit=on
  Merge : Merge
  Out1 : Outport  OutDataTypeStr=uint8
  wires:
  If/1 -> If Action Subsystem/Action
  If/2 -> If Action Subsystem1/Action
  In1/1 -> If/1
  Constant5/1 -> If Action Subsystem1/1(In1)
  Merge/1 -> Out1/1
  Constant4/1 -> If Action Subsystem/1(In1)
  If Action Subsystem/1(Out1) -> Merge/1
  If Action Subsystem1/1(Out1) -> Merge/2

== system RunningLEDExample/Subsystem6/Subsystem4 ==
  In1 : Inport
  Constant4 : Constant  Value=15  OutDataTypeStr=uint8
  Constant5 : Constant  Value=0  OutDataTypeStr=uint8
  If : If  IfExpression=u1 == 66
  If Action Subsystem : Subsystem  TreatAsAtomicUnit=on
  If Action Subsystem1 : Subsystem  TreatAsAtomicUnit=on
  Merge : Merge
  Out1 : Outport  OutDataTypeStr=uint8
  wires:
  If/1 -> If Action Subsystem/Action
  If/2 -> If Action Subsystem1/Action
  In1/1 -> If/1
  Constant5/1 -> If Action Subsystem1/1(In1)
  Merge/1 -> Out1/1
  Constant4/1 -> If Action Subsystem/1(In1)
  If Action Subsystem/1(Out1) -> Merge/1
  If Action Subsystem1/1(Out1) -> Merge/2

== system RunningLEDExample/Subsystem7/Subsystem ==
  In1 : Inport
  Constant4 : Constant  Value=15  OutDataTypeStr=uint8
  Constant5 : Constant  Value=0  OutDataTypeStr=uint8
  If : If  IfExpression=u1 == 80
  If Action Subsystem : Subsystem  TreatAsAtomicUnit=on
  If Action Subsystem1 : Subsystem  TreatAsAtomicUnit=on
  Merge : Merge
  Out1 : Outport  OutDataTypeStr=uint8
  wires:
  If/1 -> If Action Subsystem/Action
  If/2 -> If Action Subsystem1/Action
  In1/1 -> If/1
  Constant5/1 -> If Action Subsystem1/1(In1)
  Merge/1 -> Out1/1
  Constant4/1 -> If Action Subsystem/1(In1)
  If Action Subsystem/1(Out1) -> Merge/1
  If Action Subsystem1/1(Out1) -> Merge/2
